simulink model "adaptive_control"  (R2015a)
settings: Solver=ode45  StartTime=0.0  StopTime=1000  RelTol=1e-3
values from neighbouring files (symbols this model uses):
  delta = deltas(i)    [toriPlot.m]    (also in toriPlot2.m = 1)
  delta_1 = 1    [toriPlot.m]    (also in toriPlot2.m)
  delta_2 = 1    [toriPlot.m]    (also in toriPlot2.m)
  delta_3 = 1    [toriPlot.m]    (also in toriPlot2.m)
  sample_time = 0.01    [toriPlot.m]    (also in toriPlot2.m)
settings Model: Creator=ry0  LastModifiedBy=ry0

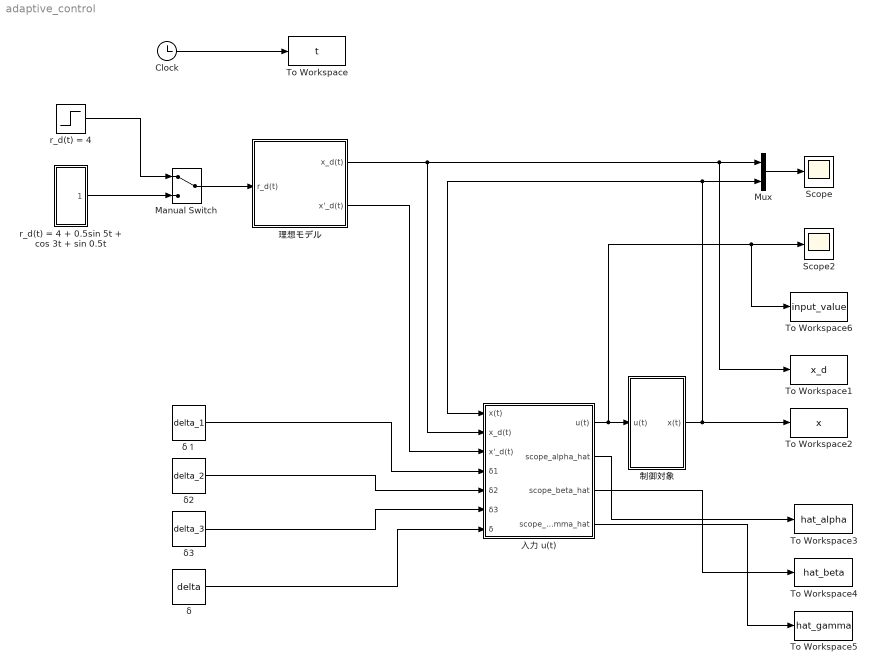
== system adaptive_control ==
  Clock : Clock
  Manual Switch : ManualSwitch
  Mux : Mux  Inputs=2
  Scope : Scope
      settings: ShowLegends=on
  Scope2 : Scope
      settings: ShowLegends=on  SaveName=ScopeData2
  To Workspace : ToWorkspace  VariableName=t  SampleTime=sample_time
  To Workspace1 : ToWorkspace  VariableName=x_d  SampleTime=sample_time
  To Workspace2 : ToWorkspace  VariableName=x  SampleTime=sample_time
  To Workspace3 : ToWorkspace  VariableName=hat_alpha  SampleTime=sample_time
  To Workspace4 : ToWorkspace  VariableName=hat_beta  SampleTime=sample_time
  To Workspace5 : ToWorkspace  VariableName=hat_gamma  SampleTime=sample_time
  To Workspace6 : ToWorkspace  VariableName=input_value  SampleTime=sample_time
  r_d(t) = 4 : Step  Time=0  After=4  SampleTime=0
  r_d(t) = 4 + 0.5sin 5t + cos 3t + sin 0.5t : Subsystem
  δ : Constant  Value=delta
  δ2 : Constant  Value=delta_2
  δ3 : Constant  Value=delta_3
  δ１ : Constant  Value=delta_1
  入力 u(t) : Subsystem
  制御対象 : Subsystem
  理想モデル : Subsystem
  wires:
  Clock/1 -> To Workspace/1
  制御対象/1(x(t)) -> To Workspace2/1, Mux/2, 入力 u(t)/1(x(t))
  理想モデル/2(x'_d(t)) -> 入力 u(t)/3(x'_d(t))
  入力 u(t)/1(u(t)) -> To Workspace6/1, Scope2/1, 制御対象/1(u(t))
  δ１/1 -> 入力 u(t)/4(δ1)
  δ2/1 -> 入力 u(t)/5(δ2)
  δ3/1 -> 入力 u(t)/6(δ3)
  δ/1 -> 入力 u(t)/7(δ)
  Mux/1 -> Scope/1
  理想モデル/1(x_d(t)) -> 入力 u(t)/2(x_d(t)), Mux/1, To Workspace1/1
  r_d(t) = 4/1 -> Manual Switch/1
  Manual Switch/1 -> 理想モデル/1(r_d(t))
  r_d(t) = 4 + 0.5sin 5t + cos 3t + sin 0.5t/1(r_d(t)) -> Manual Switch/2
  入力 u(t)/2(scope_alpha_hat) -> To Workspace3/1
  入力 u(t)/3(scope_beta_hat) -> To Workspace4/1
  入力 u(t)/4(scope_gamma_hat) -> To Workspace5/1

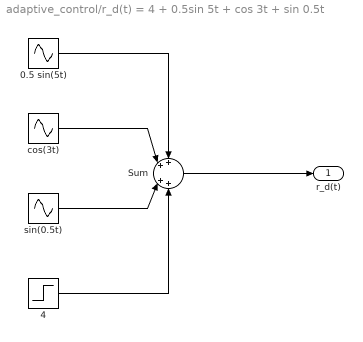
== system adaptive_control/r_d(t) = 4 + 0.5sin 5t + cos 3t + sin 0.5t ==
  0.5 sin(5t) : Sin  Amplitude=0.5  Frequency=5  SampleTime=0
  4 : Step  Time=0  After=4  SampleTime=0
  Sum : Sum  Inputs=++|++
  cos(3t) : Sin  Frequency=3  Phase=pi/2  SampleTime=0
  sin(0.5t) : Sin  Frequency=0.5  SampleTime=0
  r_d(t) : Outport
  wires:
  cos(3t)/1 -> Sum/2
  sin(0.5t)/1 -> Sum/3
  Sum/1 -> r_d(t)/1
  0.5 sin(5t)/1 -> Sum/1
  4/1 -> Sum/4

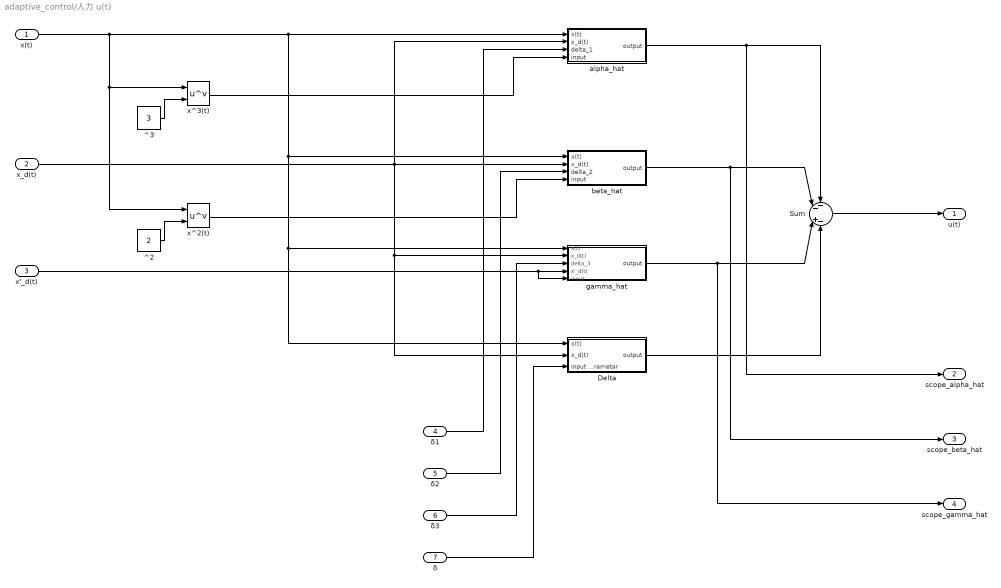
== system adaptive_control/入力 u(t) ==
  x(t) : Inport
  x_d(t) : Inport  Port=2
  x'_d(t) : Inport  Port=3
  δ1 : Inport  Port=4
  δ2 : Inport  Port=5
  δ3 : Inport  Port=6
  δ : Inport  Port=7
  Delta : Subsystem
  Sum : Sum  Inputs=--|+-
  ^2 : Constant  Value=2
  ^3 : Constant  Value=3
  alpha_hat : Subsystem
  beta_hat : Subsystem
  gamma_hat : Subsystem
  x^2(t) : Math  Operator=pow  SaturateOnIntegerOverflow=on
  x^3(t) : Math  Operator=pow  SaturateOnIntegerOverflow=on
  u(t) : Outport
  scope_alpha_hat : Outport  Port=2
  scope_beta_hat : Outport  Port=3
  scope_gamma_hat : Outport  Port=4
  wires:
  δ3/1 -> gamma_hat/3(delta_3)
  Delta/1(output) -> Sum/4
  x(t)/1 -> x^2(t)/1, x^3(t)/1, alpha_hat/1(x(t)), beta_hat/1(x(t)), gamma_hat/1(x(t)), Delta/1(x(t))
  beta_hat/1(output) -> scope_beta_hat/1, Sum/2
  x_d(t)/1 -> alpha_hat/2(x_d(t)), beta_hat/2(x_d(t)), gamma_hat/2(x_d(t)), Delta/2(x_d(t))
  x'_d(t)/1 -> gamma_hat/5(input), gamma_hat/4(x'_d(t))
  ^3/1 -> x^3(t)/2
  δ1/1 -> alpha_hat/3(delta_1)
  δ/1 -> Delta/3(Input parametar)
  ^2/1 -> x^2(t)/2
  alpha_hat/1(output) -> scope_alpha_hat/1, Sum/1
  gamma_hat/1(output) -> scope_gamma_hat/1, Sum/3
  x^3(t)/1 -> alpha_hat/4(input)
  x^2(t)/1 -> beta_hat/4(input)
  δ2/1 -> beta_hat/3(delta_2)
  Sum/1 -> u(t)/1

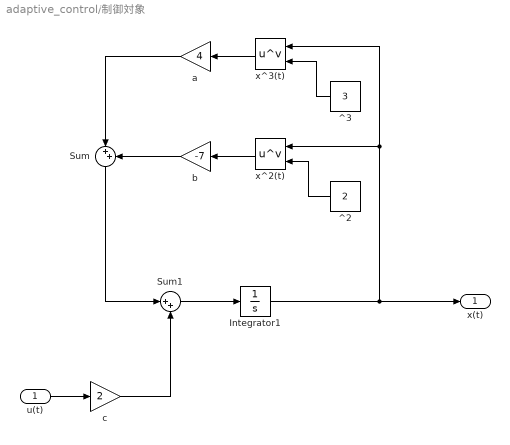
== system adaptive_control/制御対象 ==
  u(t) : Inport
  Integrator1 : Integrator
  Sum : Sum  Inputs=|++
  Sum1 : Sum  Inputs=|++
  ^2 : Constant  Value=2
  ^3 : Constant  Value=3
  a : Gain  Gain=4
  b : Gain  Gain=-7
  c : Gain  Gain=2
  x^2(t) : Math  Operator=pow  SaturateOnIntegerOverflow=on
  x^3(t) : Math  Operator=pow  SaturateOnIntegerOverflow=on
  x(t) : Outport
  wires:
  x^3(t)/1 -> a/1
  ^2/1 -> x^2(t)/2
  u(t)/1 -> c/1
  Sum1/1 -> Integrator1/1
  c/1 -> Sum1/2
  x^2(t)/1 -> b/1
  Integrator1/1 -> x(t)/1, x^2(t)/1, x^3(t)/1
  ^3/1 -> x^3(t)/2
  b/1 -> Sum/2
  a/1 -> Sum/1
  Sum/1 -> Sum1/1

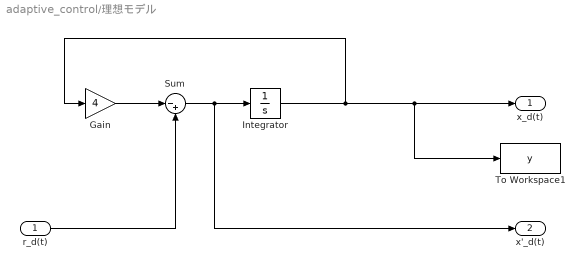
== system adaptive_control/理想モデル ==
  r_d(t) : Inport
  Gain : Gain  Gain=4
  Integrator : Integrator
  Sum : Sum  Inputs=|-+
  To Workspace1 : ToWorkspace  VariableName=y  SaveFormat=Timeseries  SampleTime=-1
  x_d(t) : Outport
  x'_d(t) : Outport  Port=2
  wires:
  Sum/1 -> x'_d(t)/1, Integrator/1
  Gain/1 -> Sum/1
  r_d(t)/1 -> Sum/2
  Integrator/1 -> x_d(t)/1, To Workspace1/1, Gain/1

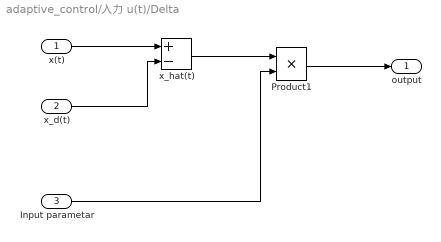
== system adaptive_control/入力 u(t)/Delta ==
  x(t) : Inport
  x_d(t) : Inport  Port=2
  Input parametar : Inport  Port=3
  Product1 : Product
  x_hat(t) : Sum  Inputs=+-
  output : Outport
  wires:
  x(t)/1 -> x_hat(t)/1
  x_d(t)/1 -> x_hat(t)/2
  x_hat(t)/1 -> Product1/1
  Product1/1 -> output/1
  Input parametar/1 -> Product1/2

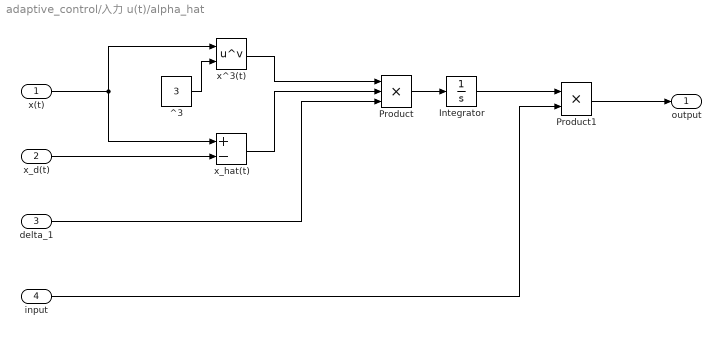
== system adaptive_control/入力 u(t)/alpha_hat ==
  x(t) : Inport
  x_d(t) : Inport  Port=2
  delta_1 : Inport  Port=3
  input : Inport  Port=4
  Integrator : Integrator
  Product : Product  Inputs=3
  Product1 : Product
  ^3 : Constant  Value=3
  x^3(t) : Math  Operator=pow  SaturateOnIntegerOverflow=on
  x_hat(t) : Sum  Inputs=+-
  output : Outport
  wires:
  x(t)/1 -> x^3(t)/1, x_hat(t)/1
  x_d(t)/1 -> x_hat(t)/2
  ^3/1 -> x^3(t)/2
  x^3(t)/1 -> Product/1
  x_hat(t)/1 -> Product/2
  delta_1/1 -> Product/3
  Product/1 -> Integrator/1
  Integrator/1 -> Product1/1
  input/1 -> Product1/2
  Product1/1 -> output/1

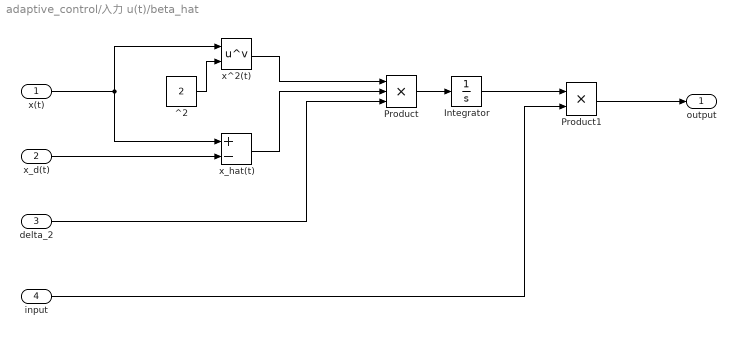
== system adaptive_control/入力 u(t)/beta_hat ==
  x(t) : Inport
  x_d(t) : Inport  Port=2
  delta_2 : Inport  Port=3
  input : Inport  Port=4
  Integrator : Integrator
  Product : Product  Inputs=3
  Product1 : Product
  ^2 : Constant  Value=2
  x^2(t) : Math  Operator=pow  SaturateOnIntegerOverflow=on
  x_hat(t) : Sum  Inputs=+-
  output : Outport
  wires:
  x(t)/1 -> x^2(t)/1, x_hat(t)/1
  x_d(t)/1 -> x_hat(t)/2
  ^2/1 -> x^2(t)/2
  x^2(t)/1 -> Product/1
  x_hat(t)/1 -> Product/2
  delta_2/1 -> Product/3
  Product/1 -> Integrator/1
  Integrator/1 -> Product1/1
  input/1 -> Product1/2
  Product1/1 -> output/1

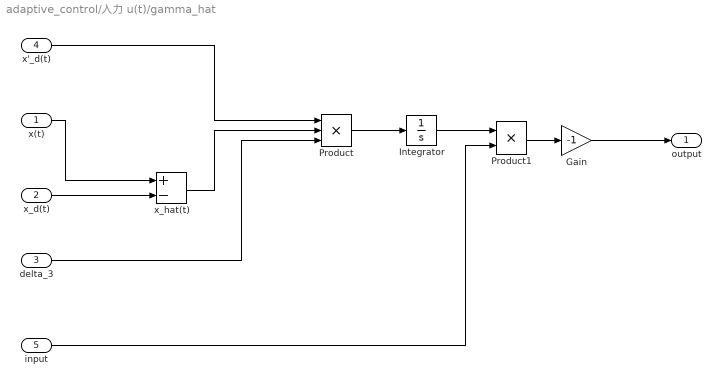
== system adaptive_control/入力 u(t)/gamma_hat ==
  x(t) : Inport
  x_d(t) : Inport  Port=2
  delta_3 : Inport  Port=3
  x'_d(t) : Inport  Port=4
  input : Inport  Port=5
  Gain : Gain  Gain=-1
  Integrator : Integrator
  Product : Product  Inputs=3
  Product1 : Product
  x_hat(t) : Sum  Inputs=+-
  output : Outport
  wires:
  x(t)/1 -> x_hat(t)/1
  x_d(t)/1 -> x_hat(t)/2
  x'_d(t)/1 -> Product/1
  x_hat(t)/1 -> Product/2
  delta_3/1 -> Product/3
  Product/1 -> Integrator/1
  Integrator/1 -> Product1/1
  input/1 -> Product1/2
  Product1/1 -> Gain/1
  Gain/1 -> output/1
